simulink model "descent_test"  (R2026a)
settings: Solver=ode23t  StopTime=100  MaxStep=0.1  RelTol=1e-4
libraries: simulink x2, fl_lib x2
settings Model: DataDictionary=scubaParams.sldd  Creator=grouleau  LastModifiedBy=grouleau

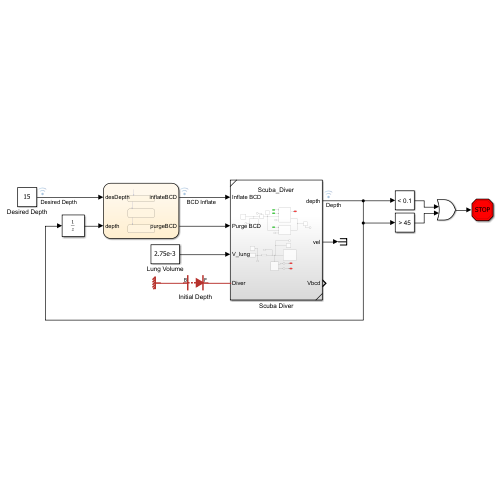
[thumbnail: Simulink's stored preview of the top-level diagram]
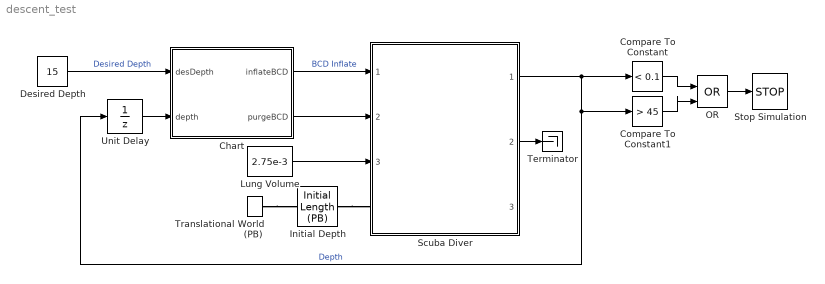
== system descent_test ==
  Chart : Stateflow chart  TreatAsAtomicUnit=on
      settings: PortSchema="{\"entries\":[{\"content\":{\"sides\":[{\"content\":{\"connectorIds\":[\"In2\",\"In1\"]},\"type\":\"ConnectorPlacement.EquallySpacedRectSide\",\"uuid\":\"e784b032-d294-47af-8dca-1d36affbd51f\"},{\"content\":{\"connectorIds\":[\"Out1\",\"Out2\"],\"side\":\"RIGHT\"},\"type\":\"ConnectorPlacement.EquallySpacedRectSide\",\"uuid\":\"b5faf6f1-96a9-41d4-9e3a-acd768d506f3\"},{\"content\":{\"side\":\"TOP\"},\"type\":\"ConnectorPlacement.EquallySpacedRectSide\",\"uuid\":\"9cb9a47b-5522-49a6-a3ce-48dfa530776a\"}]},\"type\":\"ConnectorPlacement.EquallySpacedConnector\",\"uuid\":\"608ef3a7-93ed-478d-a489-8f3c5d453485\"}],\"packageUris\":[\"http://schema.mathworks.com/mf0/Connector/R2020b\"],\"version\":\"1.0\"}"
  Compare To Constant : simulink/Logic and Bit Operations/Compare To Constant  relop=<  const=0.1  OutDataTypeStr=boolean
  Compare To Constant1 : simulink/Logic and Bit Operations/Compare To Constant  relop=>  const=45  OutDataTypeStr=boolean
  Desired Depth : Constant  Value=15  SampleTime=0.01
  Initial Depth : fl_lib/Translational/Elements/Initial Length (PB)  length_specify=on  length_priority=High  length=ic_depth m  length_nominal_specify=off  length_nominal_value=1  length_nominal_unit=m  f_specify=off  f_priority=None  f=0 N  f_nominal_specify=off  f_nominal_value=1  f_nominal_unit=N  v_rel_specify=off  v_rel_priority=None  v_rel=0 m/s  v_rel_nominal_specify=off  v_rel_nominal_value=1  v_rel_nominal_unit=m/s
  Lung Volume : Constant  Value=2.75e-3
  OR : Logic  Operator=OR  IconShape=distinctive  AllPortsSameDT=off  OutDataTypeStr=boolean
  Scuba Diver : Subsystem  ReferencedSubsystem=Scuba_Diver
  Stop Simulation : Stop
  Terminator : Terminator
  Translational World (PB) : fl_lib/Translational/Elements/Translational World (PB)
  Unit Delay : UnitDelay  InitialCondition=20  SampleTime=0.01
  wires:
  Desired Depth/1 -> Chart/2(desDepth)  "Desired Depth"
  Unit Delay/1 -> Chart/1(depth)
  Scuba Diver/1 -> Unit Delay/1, Compare To Constant1/1, Compare To Constant/1  "Depth"
  Chart/1(inflateBCD) -> Scuba Diver/1  "BCD Inflate"
  Chart/2(purgeBCD) -> Scuba Diver/2
  Scuba Diver/2 -> Terminator/1
  Lung Volume/1 -> Scuba Diver/3
  Compare To Constant/1 -> OR/1
  OR/1 -> Stop Simulation/1
  Compare To Constant1/1 -> OR/2
  connections:
  Translational World (PB)/RConn1 -- Initial Depth/LConn1
  Initial Depth/RConn1 -- Scuba Diver/LConn1

== stateflow chart descent_test/Chart ==
  state Descent
  state Inflate
    en: inflateBCD = 1;
  state Ascent
    en: inflateBCD = 0;
  (default) -> Descent : {purgeBCD = 0;}
  Descent -> Inflate : [depth >= desDepth]
  Inflate -> Ascent : after(InflateDT,sec)
  data: inflateBCD output double =0; purgeBCD output double =0; depth input; desDepth input; InflateDT parameter
